simulink model "MP7"  (R2018a)
settings: Solver=VariableStepAuto  StartTime=0.0  StopTime=10.0  RelTol=1e-3
settings Model: Creator=Halil Temurtaş  LastModifiedBy=Halil Temurtaş

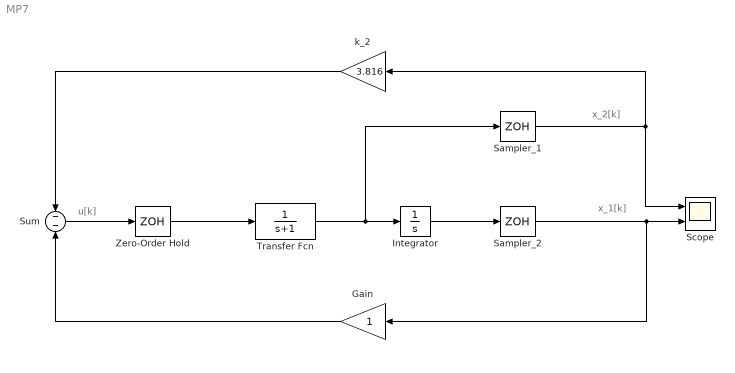
== system MP7 ==
  note: x_1[k]
  note: x_2[k]
  note: u[k]
  Gain : Gain
  Integrator : Integrator  InitialCondition=4
  Sampler_1 : ZeroOrderHold  SampleTime=-1
  Sampler_2 : ZeroOrderHold  SampleTime=-1
  Scope : Scope  NumInputPorts=2
  Sum : Sum  Inputs=--
  Transfer Fcn : TransferFcn  Denominator=[1 1]
  Zero-Order Hold : ZeroOrderHold  SampleTime=-1
  k_2 : Gain  Gain=3.816
  wires:
  Sum/1 -> Zero-Order Hold/1
  Zero-Order Hold/1 -> Transfer Fcn/1
  Transfer Fcn/1 -> Sampler_1/1, Integrator/1
  Integrator/1 -> Sampler_2/1
  Sampler_2/1 -> Gain/1, Scope/2
  Sampler_1/1 -> k_2/1, Scope/1
  Gain/1 -> Sum/2
  k_2/1 -> Sum/1
